simulink model "coord2ASV1UAV"  (R2017a)
settings: Solver=FixedStepAuto  StartTime=0.0  StopTime=720  FixedStep=0.2  RelTol=1e-3
StopFcn:
  | plotVehicles(posHist, tout, start, finish);
settings Model: Creator=acrab  LastModifiedBy=acrab

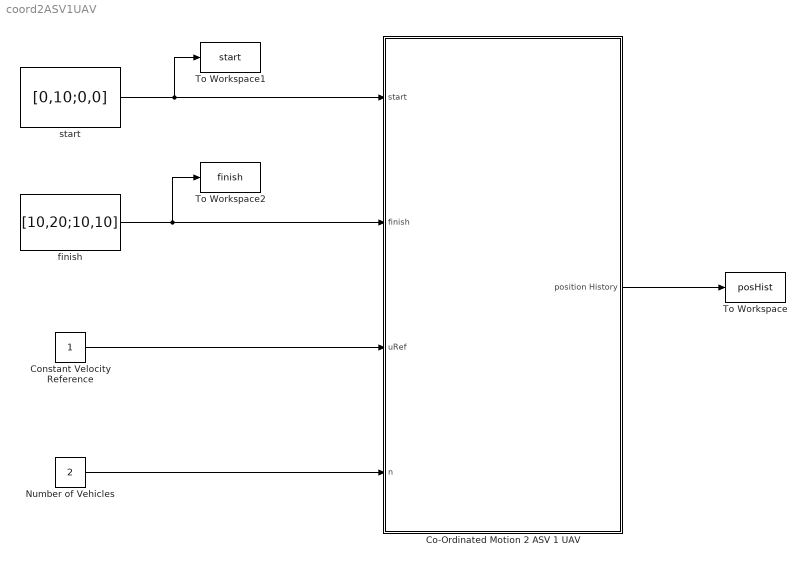
== system coord2ASV1UAV ==
  Co-Ordinated Motion 2 ASV 1 UAV : Subsystem
  Constant Velocity Reference : Constant
  Number of Vehicles : Constant  Value=2
  To Workspace : ToWorkspace  VariableName=posHist  SaveFormat=Structure With Time  SampleTime=-1
  To Workspace1 : ToWorkspace  VariableName=start  SampleTime=-1
  To Workspace2 : ToWorkspace  VariableName=finish  SampleTime=-1
  finish : Constant  Value=[10,20;10,10]
  "start " : Constant  Value=[0,10;0,0]
  wires:
  "start "/1 -> To Workspace1/1, Co-Ordinated Motion 2 ASV 1 UAV/1(start)
  finish/1 -> To Workspace2/1, Co-Ordinated Motion 2 ASV 1 UAV/2(finish)
  Constant Velocity Reference/1 -> Co-Ordinated Motion 2 ASV 1 UAV/3(uRef)
  Number of Vehicles/1 -> Co-Ordinated Motion 2 ASV 1 UAV/4(n)
  Co-Ordinated Motion 2 ASV 1 UAV/1(position History) -> To Workspace/1

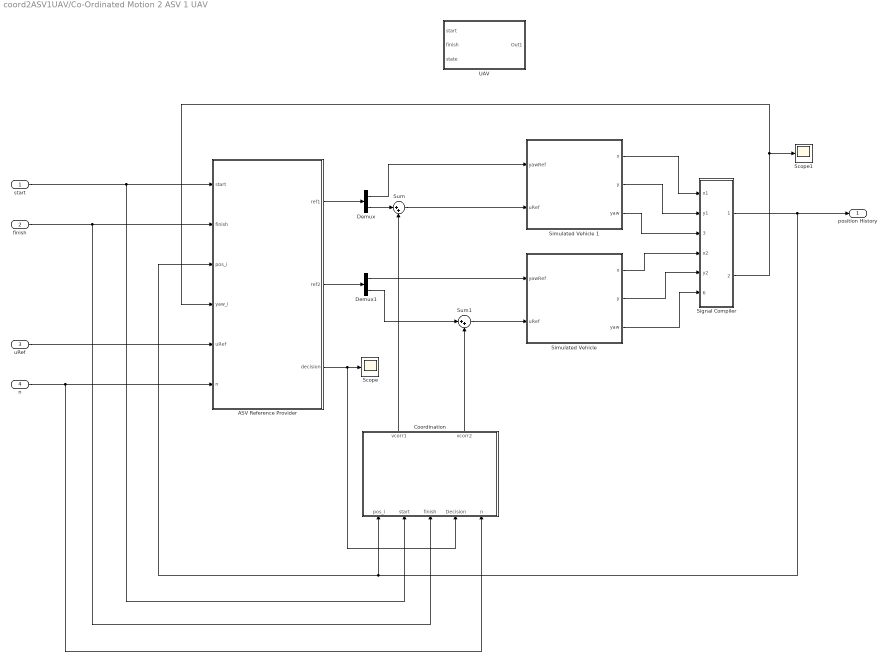
== system coord2ASV1UAV/Co-Ordinated Motion 2 ASV 1 UAV ==
  start : Inport
  finish : Inport  Port=2
  uRef : Inport  Port=3
  n : Inport  Port=4
  ASV Reference Provider : Subsystem
  Coordination : Subsystem  mask{ksync=1, ks=1}
  Demux : Demux  Outputs=2
  Demux1 : Demux  Outputs=2
  Scope : Scope
  Scope1 : Scope
  Signal Compiler : Subsystem
  Simulated Vehicle : Subsystem
  Simulated Vehicle 1 : Subsystem
  Sum : Sum  Inputs=|++
  Sum1 : Sum  Inputs=|++
  UAV : Subsystem
  position History : Outport
  wires:
  Signal Compiler/2(yaw_i) -> Scope1/1, ASV Reference Provider/4(yaw_i)
  Simulated Vehicle 1/3(yaw) -> Signal Compiler/3(yaw1)
  Simulated Vehicle/3(yaw) -> Signal Compiler/6("yaw2 ")
  Sum1/1 -> Simulated Vehicle/2(uRef)
  Demux/1 -> Simulated Vehicle 1/1(yawRef)
  Sum/1 -> Simulated Vehicle 1/2(uRef)
  Demux1/2 -> Sum1/1
  n/1 -> Coordination/5(n), ASV Reference Provider/6("n ")
  Demux1/1 -> Simulated Vehicle/1(yawRef)
  ASV Reference Provider/2("ref2 ") -> Demux1/1
  uRef/1 -> ASV Reference Provider/5(uRef)
  ASV Reference Provider/1(ref1) -> Demux/1
  Simulated Vehicle 1/2(y) -> Signal Compiler/2(y1)
  Coordination/2("vcorr2 ") -> Sum1/2
  Simulated Vehicle 1/1(x) -> Signal Compiler/1(x1)
  ASV Reference Provider/3("decision ") -> Coordination/4(Decision), Scope/1
  start/1 -> ASV Reference Provider/1(start), Coordination/2(start)
  Signal Compiler/1(pos_i) -> position History/1, Coordination/1(pos_i), ASV Reference Provider/3(pos_i)
  Coordination/1(vcorr1) -> Sum/2
  Demux/2 -> Sum/1
  Simulated Vehicle/1(x) -> Signal Compiler/4(x2)
  finish/1 -> ASV Reference Provider/2(finish), Coordination/3(finish)
  Simulated Vehicle/2(y) -> Signal Compiler/5(y2)

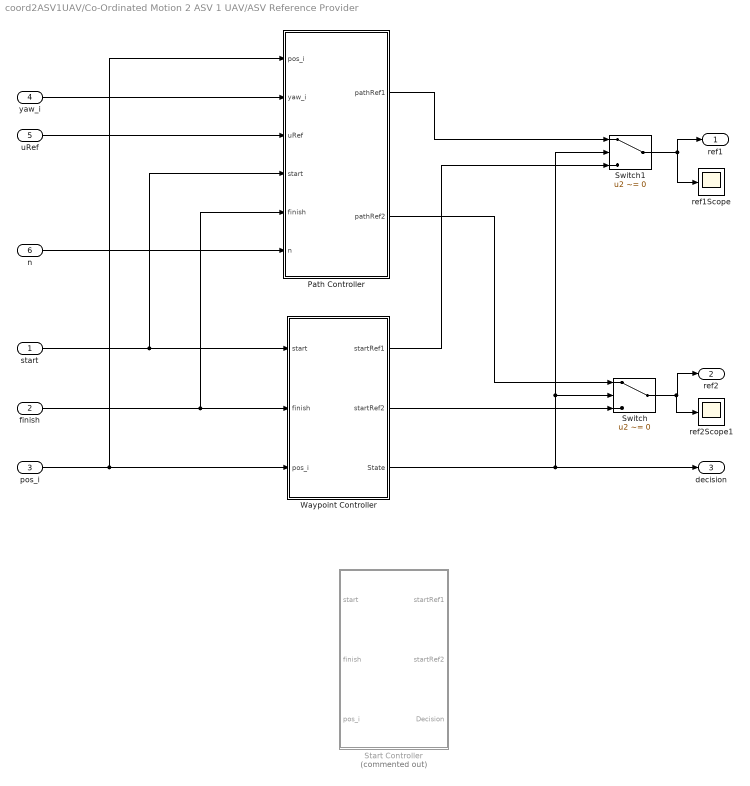
== system coord2ASV1UAV/Co-Ordinated Motion 2 ASV 1 UAV/ASV Reference Provider ==
  start : Inport
  finish : Inport  Port=2
  pos_i : Inport  Port=3
  yaw_i : Inport  Port=4
  uRef : Inport  Port=5
  "n " : Inport  Port=6
  Path Controller : Subsystem
  Start Controller : Subsystem  Commented=on  mask{ku=0.1, ks=0.1}
  Switch : Switch  Criteria=u2 ~= 0  Threshold=0.5
  Switch1 : Switch  Criteria=u2 ~= 0  Threshold=0.5
  Waypoint Controller : Subsystem  mask{ku=0.25, ks=0.1}
  ref1Scope : Scope
  ref2Scope1 : Scope
  ref1 : Outport
  "ref2 " : Outport  Port=2
  "decision " : Outport  Port=3
  wires:
  Waypoint Controller/3(State) -> Switch1/2, Switch/2, "decision "/1
  Waypoint Controller/2(startRef2) -> Switch/3
  Waypoint Controller/1(startRef1) -> Switch1/3
  Switch1/1 -> ref1Scope/1, ref1/1
  Switch/1 -> ref2Scope1/1, "ref2 "/1
  pos_i/1 -> Waypoint Controller/3(pos_i), Path Controller/1(pos_i)
  Path Controller/1(pathRef1) -> Switch1/1
  Path Controller/2(pathRef2) -> Switch/1
  yaw_i/1 -> Path Controller/2(yaw_i)
  uRef/1 -> Path Controller/3(uRef)
  start/1 -> Path Controller/4(start), Waypoint Controller/1("start ")
  finish/1 -> Waypoint Controller/2(finish), Path Controller/5(finish)
  "n "/1 -> Path Controller/6(n)

== system coord2ASV1UAV/Co-Ordinated Motion 2 ASV 1 UAV/Coordination ==
  pos_i : Inport
  start : Inport  Port=2
  finish : Inport  Port=3
  Decision : Inport  Port=4
  n : Inport  Port=5
  Co-Ordination Controller : MATLAB Function  TreatAsAtomicUnit=on
  Constant : Constant  Value=0
  vcorr1 : Outport
  "vcorr2 " : Outport  Port=2
  wires:
  n/1 -> Co-Ordination Controller/1(n)
  pos_i/1 -> Co-Ordination Controller/2(pos_i)
  start/1 -> Co-Ordination Controller/3(start)
  finish/1 -> Co-Ordination Controller/4(finish)
  Constant/1 -> Co-Ordination Controller/5(pathType)
  Co-Ordination Controller/1(vcorr1) -> vcorr1/1
  Co-Ordination Controller/2(vcorr2) -> "vcorr2 "/1
  Decision/1 -> Co-Ordination Controller/6(decision)

== system coord2ASV1UAV/Co-Ordinated Motion 2 ASV 1 UAV/Signal Compiler ==
  x1 : Inport
  y1 : Inport  Port=2
  yaw1 : Inport  Port=3
  x2 : Inport  Port=4
  y2 : Inport  Port=5
  "yaw2 " : Inport  Port=6
  MATLAB Function : MATLAB Function  TreatAsAtomicUnit=on
  pos_i : Outport
  yaw_i : Outport  Port=2
  wires:
  x2/1 -> MATLAB Function/4(x2)
  y2/1 -> MATLAB Function/5(y2)
  y1/1 -> MATLAB Function/2(y1)
  x1/1 -> MATLAB Function/1(x1)
  MATLAB Function/1(pos_i) -> pos_i/1
  yaw1/1 -> MATLAB Function/3(yaw1)
  "yaw2 "/1 -> MATLAB Function/6(yaw2)
  MATLAB Function/2(yaw_i) -> yaw_i/1

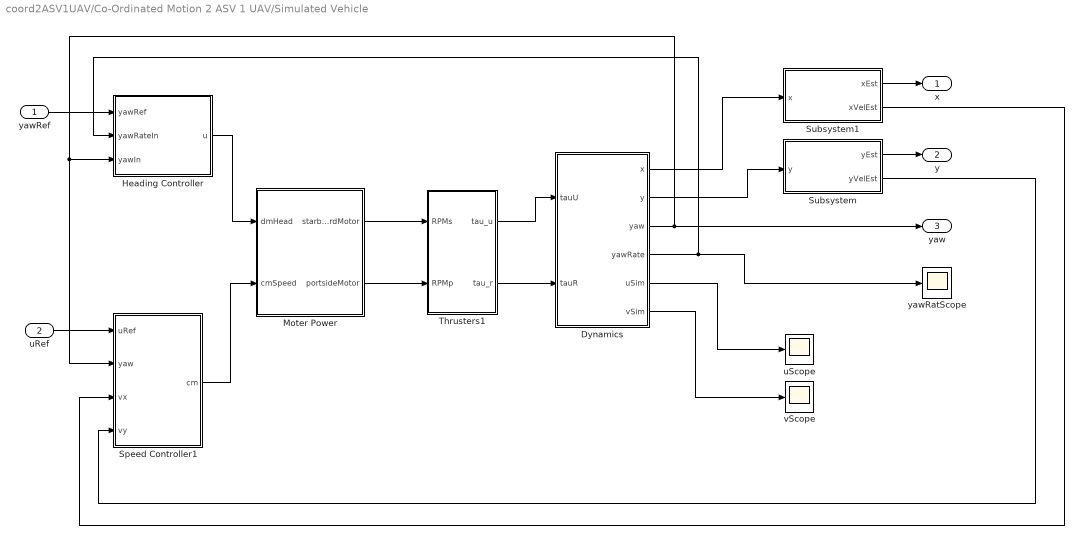
== system coord2ASV1UAV/Co-Ordinated Motion 2 ASV 1 UAV/Simulated Vehicle ==
  yawRef : Inport
  uRef : Inport  Port=2
  Dynamics : Subsystem
  Heading Controller : Subsystem  mask{Kp=45, Kd=110}
  Moter Power : Subsystem
  Speed Controller1 : Subsystem  mask{Kp=60, Ki=2, KSat=60}
      mask prompts: KSat "Saturation Level"
  Subsystem : Subsystem
  Subsystem1 : Subsystem
  Thrusters1 : Subsystem
  uScope : Scope
  vScope : Scope
  yawRatScope : Scope
  x : Outport
  y : Outport  Port=2
  yaw : Outport  Port=3
  wires:
  Thrusters1/1(tau_u) -> Dynamics/1(tauU)
  Thrusters1/2(tau_r) -> Dynamics/2(tauR)
  Moter Power/1(starboardMotor) -> Thrusters1/1(RPMs)
  Moter Power/2(portsideMotor) -> Thrusters1/2(RPMp)
  Dynamics/3(yaw) -> Speed Controller1/2(yaw), Heading Controller/3(yawIn), yaw/1
  Dynamics/4(yawRate) -> yawRatScope/1, Heading Controller/2(yawRateIn)
  Dynamics/5(uSim) -> uScope/1
  Dynamics/6(vSim) -> vScope/1
  yawRef/1 -> Heading Controller/1(yawRef)
  uRef/1 -> Speed Controller1/1(uRef)
  Subsystem/1(yEst) -> y/1
  Dynamics/2(y) -> Subsystem/1(y)
  Heading Controller/1(u) -> Moter Power/1(dmHead)
  Speed Controller1/1(cm) -> Moter Power/2(cmSpeed)
  Dynamics/1(x) -> Subsystem1/1(x)
  Subsystem1/1(xEst) -> x/1
  Subsystem/2(yVelEst) -> Speed Controller1/4(vy)
  Subsystem1/2(xVelEst) -> Speed Controller1/3(vx)

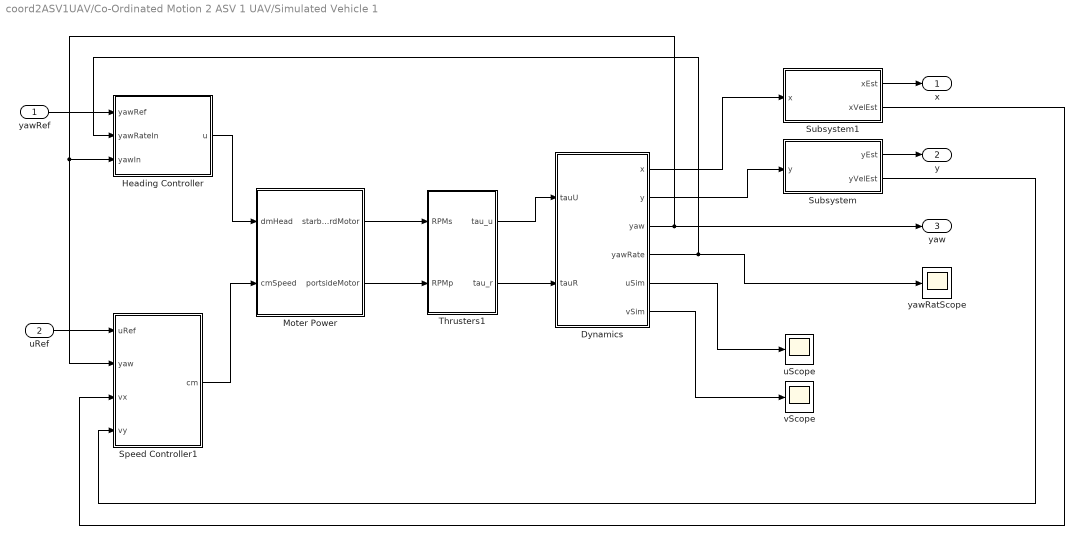
== system coord2ASV1UAV/Co-Ordinated Motion 2 ASV 1 UAV/Simulated Vehicle 1 ==
  yawRef : Inport
  uRef : Inport  Port=2
  Dynamics : Subsystem
  Heading Controller : Subsystem  mask{Kp=45, Kd=110}
  Moter Power : Subsystem
  Speed Controller1 : Subsystem  mask{Kp=60, Ki=2, KSat=60}
      mask prompts: KSat "Saturation Level"
  Subsystem : Subsystem
  Subsystem1 : Subsystem
  Thrusters1 : Subsystem
  uScope : Scope
  vScope : Scope
  yawRatScope : Scope
  x : Outport
  y : Outport  Port=2
  yaw : Outport  Port=3
  wires:
  Thrusters1/1(tau_u) -> Dynamics/1(tauU)
  Thrusters1/2(tau_r) -> Dynamics/2(tauR)
  Moter Power/1(starboardMotor) -> Thrusters1/1(RPMs)
  Moter Power/2(portsideMotor) -> Thrusters1/2(RPMp)
  Dynamics/3(yaw) -> Speed Controller1/2(yaw), Heading Controller/3(yawIn), yaw/1
  Dynamics/4(yawRate) -> yawRatScope/1, Heading Controller/2(yawRateIn)
  Dynamics/5(uSim) -> uScope/1
  Dynamics/6(vSim) -> vScope/1
  yawRef/1 -> Heading Controller/1(yawRef)
  uRef/1 -> Speed Controller1/1(uRef)
  Subsystem/1(yEst) -> y/1
  Dynamics/2(y) -> Subsystem/1(y)
  Heading Controller/1(u) -> Moter Power/1(dmHead)
  Speed Controller1/1(cm) -> Moter Power/2(cmSpeed)
  Dynamics/1(x) -> Subsystem1/1(x)
  Subsystem1/1(xEst) -> x/1
  Subsystem/2(yVelEst) -> Speed Controller1/4(vy)
  Subsystem1/2(xVelEst) -> Speed Controller1/3(vx)

== system coord2ASV1UAV/Co-Ordinated Motion 2 ASV 1 UAV/UAV ==
  start : Inport
  finish : Inport  Port=2
  state : Inport  Port=3
  Out1 : Outport

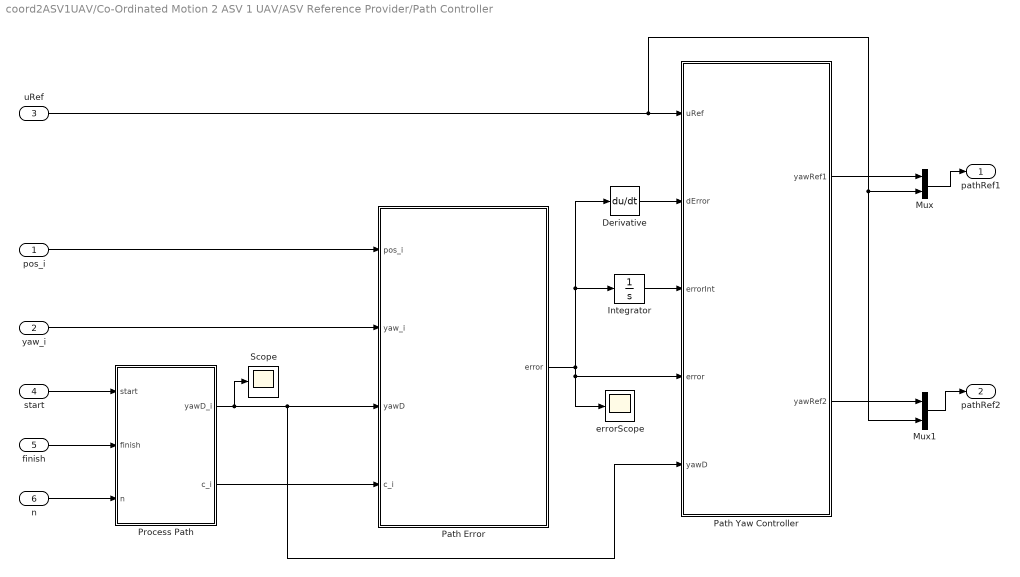
== system coord2ASV1UAV/Co-Ordinated Motion 2 ASV 1 UAV/ASV Reference Provider/Path Controller ==
  pos_i : Inport
  yaw_i : Inport  Port=2
  uRef : Inport  Port=3
  start : Inport  Port=4
  finish : Inport  Port=5
  n : Inport  Port=6
  Derivative : Derivative
  Integrator : Integrator
  Mux : Mux  Inputs=2
  Mux1 : Mux  Inputs=2
  Path Error : MATLAB Function  TreatAsAtomicUnit=on
  Path Yaw Controller : MATLAB Function  TreatAsAtomicUnit=on
  Process Path : MATLAB Function  TreatAsAtomicUnit=on
  Scope : Scope
  errorScope : Scope
  pathRef1 : Outport
  pathRef2 : Outport  Port=2
  wires:
  start/1 -> Process Path/1(start)
  Derivative/1 -> Path Yaw Controller/2(dError)
  uRef/1 -> Mux1/2, Mux/2, Path Yaw Controller/1(uRef)
  yaw_i/1 -> Path Error/2(yaw_i)
  Process Path/1(yawD_i) -> Scope/1, Path Yaw Controller/5(yawD), Path Error/3(yawD)
  Path Error/1(error) -> errorScope/1, Path Yaw Controller/4(error), Integrator/1, Derivative/1
  Process Path/2(c_i) -> Path Error/4(c_i)
  pos_i/1 -> Path Error/1(pos_i)
  n/1 -> Process Path/3(n)
  finish/1 -> Process Path/2(finish)
  Mux/1 -> pathRef1/1
  Mux1/1 -> pathRef2/1
  Path Yaw Controller/1(yawRef1) -> Mux/1
  Path Yaw Controller/2(yawRef2) -> Mux1/1
  Integrator/1 -> Path Yaw Controller/3(errorInt)

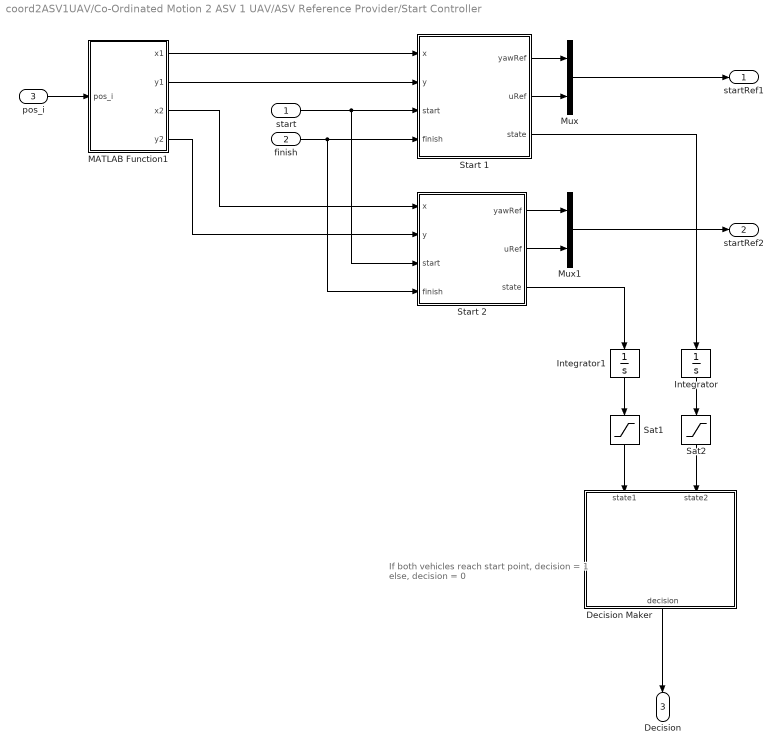
== system coord2ASV1UAV/Co-Ordinated Motion 2 ASV 1 UAV/ASV Reference Provider/Start Controller ==
  note: If both vehicles reach start point, decision = 1
      | else, decision = 0
  start : Inport
  finish : Inport  Port=2
  "pos_i " : Inport  Port=3
  Decision Maker : MATLAB Function  TreatAsAtomicUnit=on
  Integrator : Integrator
  Integrator1 : Integrator
  MATLAB Function1 : MATLAB Function  TreatAsAtomicUnit=on
  Mux : Mux  Inputs=2
  Mux1 : Mux  Inputs=2
  Sat1 : Saturate  UpperLimit=1  LowerLimit=0
  Sat2 : Saturate  UpperLimit=1  LowerLimit=0
  Start 1 : MATLAB Function  TreatAsAtomicUnit=on
  Start 2 : MATLAB Function  TreatAsAtomicUnit=on
  startRef1 : Outport
  startRef2 : Outport  Port=2
  Decision : Outport  Port=3
  wires:
  MATLAB Function1/2(y1) -> Start 1/2(y)
  start/1 -> Start 2/3(start), Start 1/3(start)
  MATLAB Function1/1(x1) -> Start 1/1(x)
  finish/1 -> Start 2/4(finish), Start 1/4(finish)
  MATLAB Function1/3(x2) -> Start 2/1(x)
  MATLAB Function1/4(y2) -> Start 2/2(y)
  Start 1/1(yawRef) -> Mux/1
  Start 1/2(uRef) -> Mux/2
  Mux/1 -> startRef1/1
  Start 2/1(yawRef) -> Mux1/1
  Start 2/2(uRef) -> Mux1/2
  Mux1/1 -> startRef2/1
  "pos_i "/1 -> MATLAB Function1/1(pos_i)
  Start 1/3(state) -> Integrator/1
  Start 2/3(state) -> Integrator1/1
  Sat1/1 -> Decision Maker/1(state1)
  Integrator1/1 -> Sat1/1
  Integrator/1 -> Sat2/1
  Sat2/1 -> Decision Maker/2(state2)
  Decision Maker/1(decision) -> Decision/1

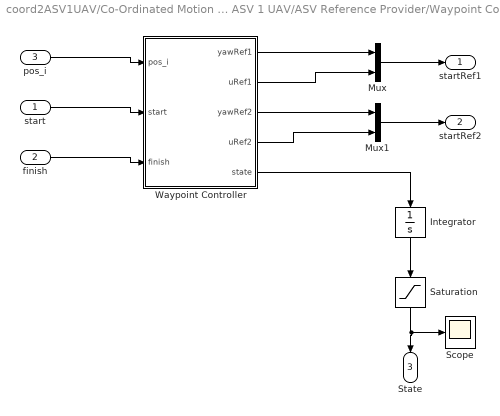
== system coord2ASV1UAV/Co-Ordinated Motion 2 ASV 1 UAV/ASV Reference Provider/Waypoint Controller ==
  "start " : Inport
  finish : Inport  Port=2
  pos_i : Inport  Port=3
  Integrator : Integrator
  Mux : Mux  Inputs=2
  Mux1 : Mux  Inputs=2
  Saturation : Saturate  UpperLimit=1  LowerLimit=0
  Scope : Scope
  Waypoint Controller : MATLAB Function  TreatAsAtomicUnit=on
  startRef1 : Outport
  startRef2 : Outport  Port=2
  State : Outport  Port=3
  wires:
  pos_i/1 -> Waypoint Controller/1(pos_i)
  "start "/1 -> Waypoint Controller/2(start)
  finish/1 -> Waypoint Controller/3(finish)
  Waypoint Controller/5(state) -> Integrator/1
  Integrator/1 -> Saturation/1
  Saturation/1 -> State/1, Scope/1
  Waypoint Controller/1(yawRef1) -> Mux/1
  Waypoint Controller/2(uRef1) -> Mux/2
  Mux/1 -> startRef1/1
  Waypoint Controller/3(yawRef2) -> Mux1/1
  Waypoint Controller/4(uRef2) -> Mux1/2
  Mux1/1 -> startRef2/1

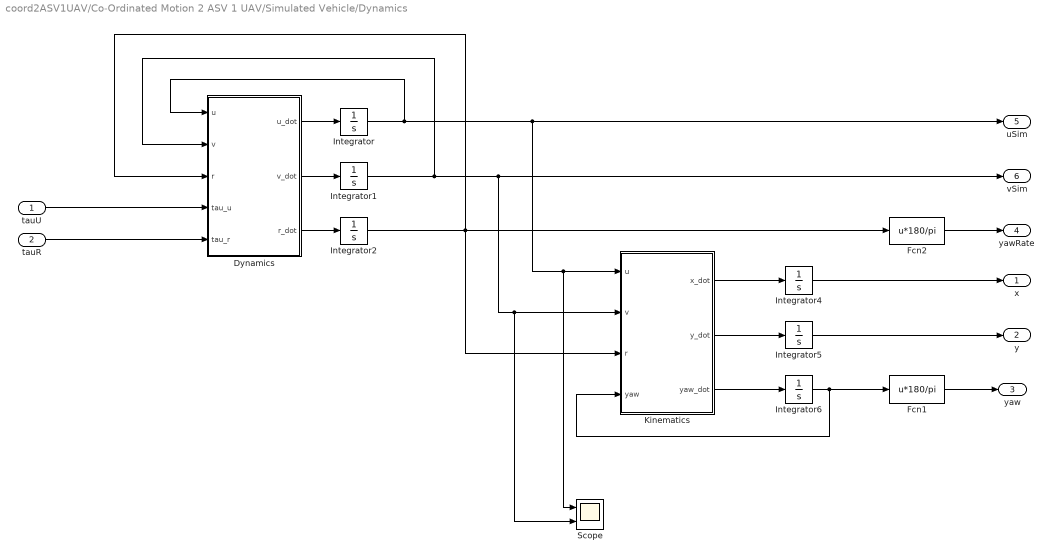
== system coord2ASV1UAV/Co-Ordinated Motion 2 ASV 1 UAV/Simulated Vehicle/Dynamics ==
  tauU : Inport
  tauR : Inport  Port=2
  Dynamics : MATLAB Function  TreatAsAtomicUnit=on
  Fcn1 : Fcn  Expr=u*180/pi
  Fcn2 : Fcn  Expr=u*180/pi
  Integrator{,1..2,4..6} (6 alike) : Integrator
  Kinematics : MATLAB Function  TreatAsAtomicUnit=on
  Scope : Scope  NumInputPorts=2
  x : Outport
  y : Outport  Port=2
  yaw : Outport  Port=3
  yawRate : Outport  Port=4
  uSim : Outport  Port=5
  vSim : Outport  Port=6
  wires:
  tauR/1 -> Dynamics/5(tau_r)
  tauU/1 -> Dynamics/4(tau_u)
  Dynamics/1(u_dot) -> Integrator/1
  Dynamics/3(r_dot) -> Integrator2/1
  Dynamics/2(v_dot) -> Integrator1/1
  Kinematics/1(x_dot) -> Integrator4/1
  Kinematics/2(y_dot) -> Integrator5/1
  Kinematics/3(yaw_dot) -> Integrator6/1
  Integrator/1 -> uSim/1, Scope/1, Kinematics/1(u), Dynamics/1(u)
  Integrator1/1 -> vSim/1, Kinematics/2(v), Scope/2, Dynamics/2(v)
  Integrator2/1 -> Fcn2/1, Kinematics/3(r), Dynamics/3(r)
  Integrator4/1 -> x/1
  Integrator5/1 -> y/1
  Integrator6/1 -> Fcn1/1, Kinematics/4(yaw)
  Fcn1/1 -> yaw/1
  Fcn2/1 -> yawRate/1

== system coord2ASV1UAV/Co-Ordinated Motion 2 ASV 1 UAV/Simulated Vehicle/Heading Controller ==
  yawRef : Inport
  yawRateIn : Inport  Port=2
  yawIn : Inport  Port=3
  Kd : Gain  Gain=Kd
  Kp : Gain  Gain=Kp
  MATLAB Function : MATLAB Function  TreatAsAtomicUnit=on
  Sum1 : Sum  Inputs=|+-
  u : Outport
  wires:
  yawRef/1 -> MATLAB Function/1(yawRef)
  yawRateIn/1 -> Kd/1
  Kd/1 -> Sum1/2
  Kp/1 -> Sum1/1
  Sum1/1 -> u/1
  MATLAB Function/1(err) -> Kp/1
  yawIn/1 -> MATLAB Function/2(yawIn)

== system coord2ASV1UAV/Co-Ordinated Motion 2 ASV 1 UAV/Simulated Vehicle/Moter Power ==
  dmHead : Inport
  cmSpeed : Inport  Port=2
  MATLAB Function : MATLAB Function  TreatAsAtomicUnit=on
  starboardMotor : Outport
  portsideMotor : Outport  Port=2
  wires:
  dmHead/1 -> MATLAB Function/1(dmHead)
  cmSpeed/1 -> MATLAB Function/2(cmSpeed)
  MATLAB Function/1(Pm) -> portsideMotor/1
  MATLAB Function/2(Sm) -> starboardMotor/1

== system coord2ASV1UAV/Co-Ordinated Motion 2 ASV 1 UAV/Simulated Vehicle/Speed Controller1 ==
  uRef : Inport
  yaw : Inport  Port=2
  vx : Inport  Port=3
  vy : Inport  Port=4
  Unit Delay : UnitDelay  SampleTime=-1
  sqr : Fcn  Expr=abs(u)*u
  u Speed from Estimates : MATLAB Function  TreatAsAtomicUnit=on
  cm : Outport
  wires:
  vx/1 -> u Speed from Estimates/1(vx)
  yaw/1 -> u Speed from Estimates/3(yaw)
  vy/1 -> u Speed from Estimates/2(vy)
  uRef/1 -> u Speed from Estimates/4(Uref)
  sqr/1 -> cm/1
  Unit Delay/1 -> u Speed from Estimates/5(intOld)
  u Speed from Estimates/1(cm) -> sqr/1
  u Speed from Estimates/2(int) -> Unit Delay/1

== system coord2ASV1UAV/Co-Ordinated Motion 2 ASV 1 UAV/Simulated Vehicle/Subsystem ==
  y : Inport
  Derivative : Derivative
  yEst : Outport
  yVelEst : Outport  Port=2
  wires:
  y/1 -> Derivative/1, yEst/1
  Derivative/1 -> yVelEst/1

== system coord2ASV1UAV/Co-Ordinated Motion 2 ASV 1 UAV/Simulated Vehicle/Subsystem1 ==
  x : Inport
  Derivative : Derivative
  xEst : Outport
  xVelEst : Outport  Port=2
  wires:
  x/1 -> Derivative/1, xEst/1
  Derivative/1 -> xVelEst/1

== system coord2ASV1UAV/Co-Ordinated Motion 2 ASV 1 UAV/Simulated Vehicle/Thrusters1 ==
  RPMs : Inport
  RPMp : Inport  Port=2
  Add : Sum
  Add1 : Sum  Inputs=-+
  Motor Port : Subsystem  mask{K0=7.2115, tau=0.346, eta=4/(1500^2)}
      mask prompts: tau "Atraso do Motor"; eta "Constante de conversao W-F"
  Motor Stardboard : Subsystem  mask{K0=7.2115, tau=0.346, eta=4/(1500^2)}
      mask prompts: tau "Atraso do Motor"; eta "Constante de conversao W-F"
  l : Gain  Gain=0.25
  tau_u : Outport
  tau_r : Outport  Port=2
  wires:
  Add1/1 -> l/1
  RPMs/1 -> Motor Stardboard/1(w RPM)
  Add/1 -> tau_u/1
  RPMp/1 -> Motor Port/1(w RPM)
  l/1 -> tau_r/1
  Motor Port/1(F) -> Add/2, Add1/2
  Motor Stardboard/1(F) -> Add/1, Add1/1

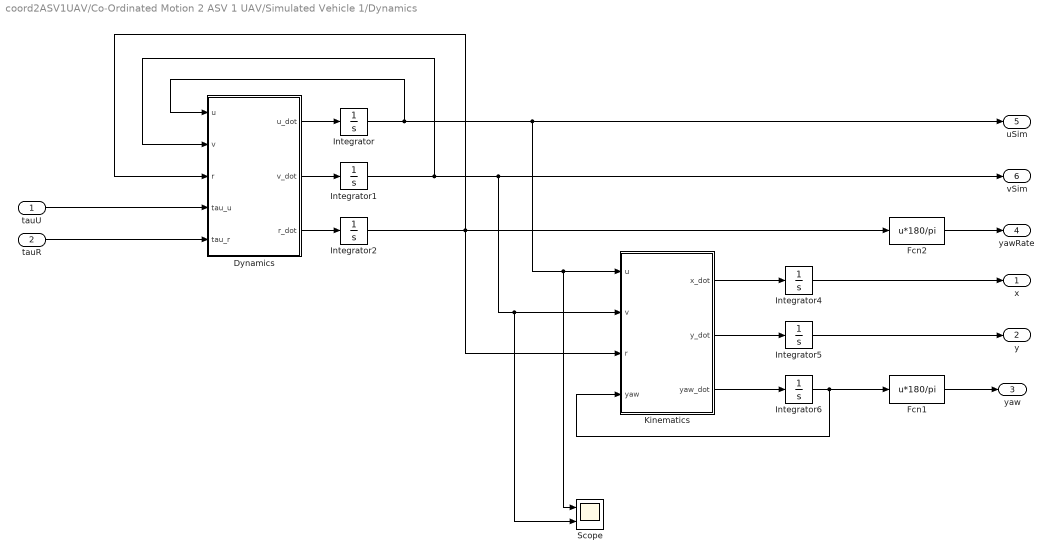
== system coord2ASV1UAV/Co-Ordinated Motion 2 ASV 1 UAV/Simulated Vehicle 1/Dynamics ==
  tauU : Inport
  tauR : Inport  Port=2
  Dynamics : MATLAB Function  TreatAsAtomicUnit=on
  Fcn1 : Fcn  Expr=u*180/pi
  Fcn2 : Fcn  Expr=u*180/pi
  Integrator{,1..2,4..6} (6 alike) : Integrator
  Kinematics : MATLAB Function  TreatAsAtomicUnit=on
  Scope : Scope  NumInputPorts=2
  x : Outport
  y : Outport  Port=2
  yaw : Outport  Port=3
  yawRate : Outport  Port=4
  uSim : Outport  Port=5
  vSim : Outport  Port=6
  wires:
  tauR/1 -> Dynamics/5(tau_r)
  tauU/1 -> Dynamics/4(tau_u)
  Dynamics/1(u_dot) -> Integrator/1
  Dynamics/3(r_dot) -> Integrator2/1
  Dynamics/2(v_dot) -> Integrator1/1
  Kinematics/1(x_dot) -> Integrator4/1
  Kinematics/2(y_dot) -> Integrator5/1
  Kinematics/3(yaw_dot) -> Integrator6/1
  Integrator/1 -> uSim/1, Scope/1, Kinematics/1(u), Dynamics/1(u)
  Integrator1/1 -> vSim/1, Kinematics/2(v), Scope/2, Dynamics/2(v)
  Integrator2/1 -> Fcn2/1, Kinematics/3(r), Dynamics/3(r)
  Integrator4/1 -> x/1
  Integrator5/1 -> y/1
  Integrator6/1 -> Fcn1/1, Kinematics/4(yaw)
  Fcn1/1 -> yaw/1
  Fcn2/1 -> yawRate/1

== system coord2ASV1UAV/Co-Ordinated Motion 2 ASV 1 UAV/Simulated Vehicle 1/Heading Controller ==
  yawRef : Inport
  yawRateIn : Inport  Port=2
  yawIn : Inport  Port=3
  Kd : Gain  Gain=Kd
  Kp : Gain  Gain=Kp
  MATLAB Function : MATLAB Function  TreatAsAtomicUnit=on
  Sum1 : Sum  Inputs=|+-
  u : Outport
  wires:
  yawRef/1 -> MATLAB Function/1(yawRef)
  yawRateIn/1 -> Kd/1
  Kd/1 -> Sum1/2
  Kp/1 -> Sum1/1
  Sum1/1 -> u/1
  MATLAB Function/1(err) -> Kp/1
  yawIn/1 -> MATLAB Function/2(yawIn)

== system coord2ASV1UAV/Co-Ordinated Motion 2 ASV 1 UAV/Simulated Vehicle 1/Moter Power ==
  dmHead : Inport
  cmSpeed : Inport  Port=2
  MATLAB Function : MATLAB Function  TreatAsAtomicUnit=on
  starboardMotor : Outport
  portsideMotor : Outport  Port=2
  wires:
  dmHead/1 -> MATLAB Function/1(dmHead)
  cmSpeed/1 -> MATLAB Function/2(cmSpeed)
  MATLAB Function/1(Pm) -> portsideMotor/1
  MATLAB Function/2(Sm) -> starboardMotor/1

== system coord2ASV1UAV/Co-Ordinated Motion 2 ASV 1 UAV/Simulated Vehicle 1/Speed Controller1 ==
  uRef : Inport
  yaw : Inport  Port=2
  vx : Inport  Port=3
  vy : Inport  Port=4
  Unit Delay : UnitDelay  SampleTime=-1
  sqr : Fcn  Expr=abs(u)*u
  u Speed from Estimates : MATLAB Function  TreatAsAtomicUnit=on
  cm : Outport
  wires:
  vx/1 -> u Speed from Estimates/1(vx)
  yaw/1 -> u Speed from Estimates/3(yaw)
  vy/1 -> u Speed from Estimates/2(vy)
  uRef/1 -> u Speed from Estimates/4(Uref)
  sqr/1 -> cm/1
  Unit Delay/1 -> u Speed from Estimates/5(intOld)
  u Speed from Estimates/1(cm) -> sqr/1
  u Speed from Estimates/2(int) -> Unit Delay/1

== system coord2ASV1UAV/Co-Ordinated Motion 2 ASV 1 UAV/Simulated Vehicle 1/Subsystem ==
  y : Inport
  Derivative : Derivative
  yEst : Outport
  yVelEst : Outport  Port=2
  wires:
  y/1 -> Derivative/1, yEst/1
  Derivative/1 -> yVelEst/1

== system coord2ASV1UAV/Co-Ordinated Motion 2 ASV 1 UAV/Simulated Vehicle 1/Subsystem1 ==
  x : Inport
  Derivative : Derivative
  xEst : Outport
  xVelEst : Outport  Port=2
  wires:
  x/1 -> Derivative/1, xEst/1
  Derivative/1 -> xVelEst/1

== system coord2ASV1UAV/Co-Ordinated Motion 2 ASV 1 UAV/Simulated Vehicle 1/Thrusters1 ==
  RPMs : Inport
  RPMp : Inport  Port=2
  Add : Sum
  Add1 : Sum  Inputs=-+
  Motor Port : Subsystem  mask{K0=7.2115, tau=0.346, eta=4/(1500^2)}
      mask prompts: tau "Atraso do Motor"; eta "Constante de conversao W-F"
  Motor Stardboard : Subsystem  mask{K0=7.2115, tau=0.346, eta=4/(1500^2)}
      mask prompts: tau "Atraso do Motor"; eta "Constante de conversao W-F"
  l : Gain  Gain=0.25
  tau_u : Outport
  tau_r : Outport  Port=2
  wires:
  Add1/1 -> l/1
  RPMs/1 -> Motor Stardboard/1(w RPM)
  Add/1 -> tau_u/1
  RPMp/1 -> Motor Port/1(w RPM)
  l/1 -> tau_r/1
  Motor Port/1(F) -> Add/2, Add1/2
  Motor Stardboard/1(F) -> Add/1, Add1/1

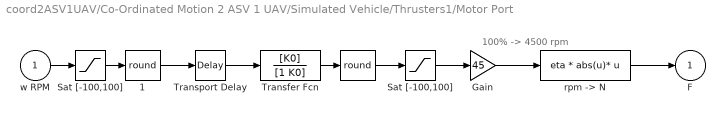
== system coord2ASV1UAV/Co-Ordinated Motion 2 ASV 1 UAV/Simulated Vehicle/Thrusters1/Motor Port ==
  note: 100% -> 4500 rpm
  w RPM : Inport
  "  " : Rounding  Operator=round
  "  1" : Rounding  Operator=round
  Gain : Gain  Gain=45
  Sat [-100,100] : Saturate  UpperLimit=100  LowerLimit=-100
  "Sat [-100,100] " : Saturate  UpperLimit=100  LowerLimit=-100
  Transfer Fcn : TransferFcn  Numerator=[K0]  Denominator=[1 K0]
  Transport Delay : TransportDelay  DelayTime=tau
  "rpm -> N" : Fcn  Expr=eta * abs(u)* u
  F : Outport
  wires:
  Transfer Fcn/1 -> "  "/1
  Transport Delay/1 -> Transfer Fcn/1
  "  1"/1 -> Transport Delay/1
  "  "/1 -> "Sat [-100,100] "/1
  "rpm -> N"/1 -> F/1
  Sat [-100,100]/1 -> "  1"/1
  Gain/1 -> "rpm -> N"/1
  w RPM/1 -> Sat [-100,100]/1
  "Sat [-100,100] "/1 -> Gain/1

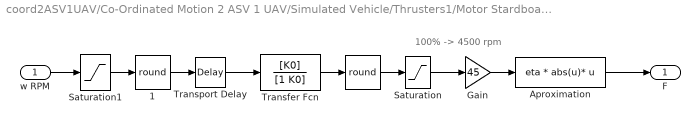
== system coord2ASV1UAV/Co-Ordinated Motion 2 ASV 1 UAV/Simulated Vehicle/Thrusters1/Motor Stardboard ==
  note: 100% -> 4500 rpm
  w RPM : Inport
  "  " : Rounding  Operator=round
  "  1" : Rounding  Operator=round
  Aproximation : Fcn  Expr=eta * abs(u)* u
  Gain : Gain  Gain=45
  Saturation : Saturate  UpperLimit=100  LowerLimit=-100
  Saturation1 : Saturate  UpperLimit=100  LowerLimit=-100
  Transfer Fcn : TransferFcn  Numerator=[K0]  Denominator=[1 K0]
  Transport Delay : TransportDelay  DelayTime=tau
  F : Outport
  wires:
  Transfer Fcn/1 -> "  "/1
  Transport Delay/1 -> Transfer Fcn/1
  "  1"/1 -> Transport Delay/1
  "  "/1 -> Saturation/1
  Aproximation/1 -> F/1
  Saturation1/1 -> "  1"/1
  Gain/1 -> Aproximation/1
  w RPM/1 -> Saturation1/1
  Saturation/1 -> Gain/1

== system coord2ASV1UAV/Co-Ordinated Motion 2 ASV 1 UAV/Simulated Vehicle 1/Thrusters1/Motor Port ==
  note: 100% -> 4500 rpm
  w RPM : Inport
  "  " : Rounding  Operator=round
  "  1" : Rounding  Operator=round
  Gain : Gain  Gain=45
  Sat [-100,100] : Saturate  UpperLimit=100  LowerLimit=-100
  "Sat [-100,100] " : Saturate  UpperLimit=100  LowerLimit=-100
  Transfer Fcn : TransferFcn  Numerator=[K0]  Denominator=[1 K0]
  Transport Delay : TransportDelay  DelayTime=tau
  "rpm -> N" : Fcn  Expr=eta * abs(u)* u
  F : Outport
  wires:
  Transfer Fcn/1 -> "  "/1
  Transport Delay/1 -> Transfer Fcn/1
  "  1"/1 -> Transport Delay/1
  "  "/1 -> "Sat [-100,100] "/1
  "rpm -> N"/1 -> F/1
  Sat [-100,100]/1 -> "  1"/1
  Gain/1 -> "rpm -> N"/1
  w RPM/1 -> Sat [-100,100]/1
  "Sat [-100,100] "/1 -> Gain/1

== system coord2ASV1UAV/Co-Ordinated Motion 2 ASV 1 UAV/Simulated Vehicle 1/Thrusters1/Motor Stardboard ==
  note: 100% -> 4500 rpm
  w RPM : Inport
  "  " : Rounding  Operator=round
  "  1" : Rounding  Operator=round
  Aproximation : Fcn  Expr=eta * abs(u)* u
  Gain : Gain  Gain=45
  Saturation : Saturate  UpperLimit=100  LowerLimit=-100
  Saturation1 : Saturate  UpperLimit=100  LowerLimit=-100
  Transfer Fcn : TransferFcn  Numerator=[K0]  Denominator=[1 K0]
  Transport Delay : TransportDelay  DelayTime=tau
  F : Outport
  wires:
  Transfer Fcn/1 -> "  "/1
  Transport Delay/1 -> Transfer Fcn/1
  "  1"/1 -> Transport Delay/1
  "  "/1 -> Saturation/1
  Aproximation/1 -> F/1
  Saturation1/1 -> "  1"/1
  Gain/1 -> Aproximation/1
  w RPM/1 -> Saturation1/1
  Saturation/1 -> Gain/1

== matlab function coord2ASV1UAV/Co-Ordinated Motion 2 ASV 1 UAV/Simulated Vehicle 1/Dynamics/Dynamics ==
  data: u input; u_dot output; v input; r input; tau_u input; tau_r input; v_dot output; r_dot output
function [u_dot,v_dot,r_dot] = fcn(u,v,r,tau_u,tau_r)

% Coefficients
m = 17; %kg
Iz = 1; %4.14;
X_u_dot = -20;
Y_v_dot = -30;%-1.3175;
N_r_dot = -8.69;% -0.5;
X_u = -0.2;
Y_v = -50; %-55.117;
N_r = -4.14; %-0.1
X_uu = -25;
Y_vv = -0.01;%-101.2776;
N_rr = -6.23; %-21

% Added Mass
mu = m - X_u_dot;
mv = m - Y_v_dot;
mr = Iz - N_r_dot;
muv = mu - mv;

% Hydrodynamic Damping
du = - X_u - X_uu*abs(u);
dv = - Y_v - Y_vv*abs(v);
dr = - N_r - N_rr*abs(r);

% State Derivatives
u_dot = 1/mu*(tau_u + mv*v*r - du*u);
v_dot = 1/mv*(- mu*u*r - dv*v);
r_dot = 1/mr*(tau_r + muv*u*v - dr*r);

== matlab function coord2ASV1UAV/Co-Ordinated Motion 2 ASV 1 UAV/Simulated Vehicle 1/Speed Controller1/u Speed from Estimates ==
  data: vx input; cm output; vy input; yaw input; Uref input; int output; intOld input; Kp parameter; Ki parameter; KSat parameter
function [cm,int] = ExtractSpeed(vx,vy,yaw,Uref,intOld,Kp, Ki, KSat)

% Kp = 60;
% Ki = 2;
% KSat = 60;
 
u = vx*sind(yaw) + vy*cosd(yaw);
err = u - Uref;
int = intOld + err;

cm = - Kp*err - Ki*int;

if(abs(cm) >= KSat)
   cm = KSat*sign(cm); 
   int = intOld;
end

== matlab function coord2ASV1UAV/Co-Ordinated Motion 2 ASV 1 UAV/Simulated Vehicle 1/Dynamics/Kinematics ==
  data: u input; x_dot output; v input; r input; yaw input; y_dot output; yaw_dot output
function [x_dot,y_dot,yaw_dot] = fcn(u,v,r,yaw)

y_dot = u*cos(yaw) - v*sin(yaw);
x_dot = u*sin(yaw) + v*cos(yaw);
yaw_dot = r;

== matlab function coord2ASV1UAV/Co-Ordinated Motion 2 ASV 1 UAV/Simulated Vehicle 1/Moter Power/MATLAB Function ==
  data: dmHead input; cmSpeed input; Pm output; Sm output
function [Pm,Sm] = fcn(dmHead,cmSpeed)

Cm_sqr = cmSpeed;
Dm_sqr = dmHead;

Pm = round(sqrt(abs(Cm_sqr+Dm_sqr))*sign(Cm_sqr+Dm_sqr));
Sm = round(sqrt(abs(Cm_sqr-Dm_sqr))*sign(Cm_sqr-Dm_sqr));

== matlab function coord2ASV1UAV/Co-Ordinated Motion 2 ASV 1 UAV/Simulated Vehicle 1/Heading Controller/MATLAB Function ==
  data: err output; yawRef input; yawIn input
function err = fcn(yawRef,yawIn)
%error term
err = yawRef - yawIn;

%normalize
if(err>180) 
     err = err - 360; 
elseif(err<-180)   
     err = 360 + err;
     
end

== matlab function coord2ASV1UAV/Co-Ordinated Motion 2 ASV 1 UAV/Simulated Vehicle/Dynamics/Dynamics ==
  data: u input; u_dot output; v input; r input; tau_u input; tau_r input; v_dot output; r_dot output
function [u_dot,v_dot,r_dot] = fcn(u,v,r,tau_u,tau_r)

% Coefficients
m = 17; %kg
Iz = 1; %4.14;
X_u_dot = -20;
Y_v_dot = -30;%-1.3175;
N_r_dot = -8.69;% -0.5;
X_u = -0.2;
Y_v = -50; %-55.117;
N_r = -4.14; %-0.1
X_uu = -25;
Y_vv = -0.01;%-101.2776;
N_rr = -6.23; %-21

% Added Mass
mu = m - X_u_dot;
mv = m - Y_v_dot;
mr = Iz - N_r_dot;
muv = mu - mv;

% Hydrodynamic Damping
du = - X_u - X_uu*abs(u);
dv = - Y_v - Y_vv*abs(v);
dr = - N_r - N_rr*abs(r);

% State Derivatives
u_dot = 1/mu*(tau_u + mv*v*r - du*u);
v_dot = 1/mv*(- mu*u*r - dv*v);
r_dot = 1/mr*(tau_r + muv*u*v - dr*r);

== matlab function coord2ASV1UAV/Co-Ordinated Motion 2 ASV 1 UAV/ASV Reference Provider/Path Controller/Path Yaw Controller ==
  data: yawRef1 output; uRef input; dError input; errorInt input; error input; yawRef2 output; yawD input
function [yawRef1, yawRef2]  = yawController(uRef, dError, errorInt, error, yawD)
%number of vehicles
n = 2;

% Gain Values
K1 =  6.0; %yaw proportional
K2 =  10.0; %cross-track proportional
K3 =  0.0; %cross-track differential
K4 =  0.6; %integral

%assign matrices
yawDel = zeros(1,n);

    %loop through vehicles
    for i = 1:n
        %extract data
        yError     =    error(1,i);
        yawError   =    error(2,i);
        yError_dot =   dError(1,i);
        yInt       = errorInt(1,i);

        %provide delta term
        yawDel(1,i) = K1*yawError + K2*yError/uRef ...
                      + K3*yError_dot + K4*yInt;
    end   
    
%provide yawRef values (2 VEHICLES)
yawRef1 = + yawDel(1,1) + yawD(1,1);
yawRef2 = + yawDel(1,2) + yawD(1,2);

end

== matlab function coord2ASV1UAV/Co-Ordinated Motion 2 ASV 1 UAV/ASV Reference Provider/Path Controller/Process Path ==
  data: start input; yawD_i output; c_i output; finish input; n input
function [yawD_i, c_i] = fcn(start, finish ,n)
% INPUTS
% n     = vehicle ID no.
% start = [xs1, xs2,...,xsi;
%          ys1, ys2,...,ysi]
% end   = [xe1, xe2,...,xei;
%          ye1, ye2,...,yei]
% for i = {1,..,n} vehicles


% % desired yaw
% m1 = (finish(2,1) - start(2,1)) / (finish(1,1) - start(1,1));
% m2 = (finish(2,2) - start(2,2)) / (finish(1,2) - start(1,2));
% yawD1 = atand(m1);
% yawD2 = atand(m2);
% yawD_i = [yawD1, yawD2];
% 
% % y intercept
% c1 = start(2,1) - m1*start(1,1);
% c2 = start(2,2) - m2*start(1,2);
% c_i = [c1, c2];

n = 2;

%assign matrices
yawD_i = zeros(1,n);
c_i    = zeros(1,n);

%loop through vehicles
for i = 1:n

    %desired yaw
    m = (finish(2,i) - start(2,i)) / (finish(1,i) - start(1,i));
    yawD_i(1,i) = -atan2d((finish(2,i) - start(2,i)),(finish(1,i) - start(1,i))) + 90;

    %y intersection
    c_i(1,i)    = start(2,i) - m*start(1,i);
end
end

== matlab function coord2ASV1UAV/Co-Ordinated Motion 2 ASV 1 UAV/ASV Reference Provider/Path Controller/Path Error ==
  data: pos_i input; yaw_i input; yawD input; c_i input; error output
% ========================================= %
% Calculating the cross track error between %
% defined path line and current position    %
% ========================================= %

function error  = pathError(pos_i, yaw_i, yawD, c_i)

% ARGUMENTS %
% x          current x position
% y          current y position
% m          gradient (for y = mx + c)
% c          y offset (for y = mx + c)

% VARIABLES %
% xD, yD     closest points on line
% error      error in [x, y, yaw]'
% u          vector between desired and real paths 

%number of vehicles
n = 2;

%assign matrices
error    = zeros(2,n);

%function to minimize
    function u = lineDiff(xL)
        u = (xL - x)^2 + (m*xL + c - y)^2;
    end

%loop through vehicles
for i = 1:n
    
    %extract data
    x = pos_i(1,i);
    y = pos_i(2,i);
    m = tand(-yawD(1,i) + 90);
    if (abs(m) == Inf)
        m = 1000000;
    end
    c = c_i(1,i);    
    
    %desired position
    xD = fminbnd(@lineDiff,x-10,x+10);
    yD = m*xD + c;
    closestPoint = [xD,yD];

    %cross track error
%     e = sqrt(lineDiff(xD));
    e = sqrt((xD-x)^2 + (yD - y)^2);
    if y < (m*x + c)
        e = -e;
    end

    %yaw error
    yawErr = + yawD(1,i) - yaw_i(1,i);

    %combine error terms
    error(1,i) = e;
    error(2,i) = yawErr;

end
end

== matlab function coord2ASV1UAV/Co-Ordinated Motion 2 ASV 1 UAV/ASV Reference Provider/Start Controller/Decision Maker ==
  data: state1 input; decision output; state2 input
function decision = fcn(state1, state2)
% If both vehicles reach start point, decision = 1
    if (state1 > 0 && state2 > 0)
        decision = 1;
    else
        decision = 0;
    end
end

== matlab function coord2ASV1UAV/Co-Ordinated Motion 2 ASV 1 UAV/ASV Reference Provider/Start Controller/Start 1 ==
  data: yawRef output; x input; y input; uRef output; start input; finish input; ku parameter; ks parameter; state output
% % % START POINT CONTROLLER % % %
% Make vehicle reach desired point
% Orient vehicle in direction of path

function [yawRef, uRef, state] = wayPoint(x,y, start, finish, ku, ks)
    % Go to waypoint
    state = 0;

    % Margin of error
    e = 0.1;

    % Extract information from inputs
    point1 =  start(:,1);
    point2 = finish(:,1);

    xd1 = point1(1,1);
    yd1 = point1(2,1);

    xd2 = point2(1,1);
    yd2 = point2(2,1);

    % Distance to waypoint
    d = sqrt((x - xd1)^2 + (y - yd1)^2) - e;

    % Decide on action
    if (d < 0) % vehicle in desired region
        state = 1;
        uRef = 0;
        % point in direction of path
        yawRef = -atan2d((yd2-yd1),(xd2-xd1)) + 90;
    else % vehicle outwith region
        uRef = ku*asin(d /(abs(d)+ks))*2/pi;
        yawRef = -atan2d((yd1-y), (xd1-x)) + 90;
    end
end

== matlab function coord2ASV1UAV/Co-Ordinated Motion 2 ASV 1 UAV/Coordination/Co-Ordination Controller ==
  data: n input; vcorr1 output; pos_i input size=[2,2]; start input; finish input; pathType input; vcorr2 output; ks parameter; ksync parameter; decision input
%% COORDINATION CONTROLLER
% ----INPUTS---- %
% VEHICLES
%  n = number of vehicles

% CURRENT STATE
% pos_i    = [x1, x2, ..., xn;
%             y1, y2, ..., yn];
% where i  = {1,n}
% decision = 1 ; if coordination required
% decision = 0 ; otherwise

% PATH DEFINITION
% point = [xs1, xs2, ..., xsn;
%          ys1, ys2, ..., ysn];
% where s is start, f is finish
% number denotes vehicle number
%
% pathType
% 0: line
% 1: arc

% ----OUTPUT---- %
% vcorr = [vcorr1, vcorr2, ..., vcorrn] (m/s)
%% IMPLEMENTATION
function [vcorr1,vcorr2]  = coOrd(n, pos_i, start, finish, pathType, ks, ksync, decision)
% Check whether in path following mode
if decision > 0
    % Check inputs valid
    [a,b] = size(start);
    [c,d] = size(finish);
    if (a ~= 2 || b ~= n || c ~= 2 || d ~= n )
        disp('path variable invalid')
    end

    % establish matrice sizes
    gamma  = zeros(1,n);
    gammaE = zeros(1,n);
    vcorr  = zeros(1,n);
    length = zeros(1,n);

    % CALCULATE PATH LENGTH VARIABLES
    switch pathType
        % STRAIGHT LINE
        case 0
            for i = 1:n
                length(1,i) = sqrt((finish(1,i)-start(1,i))^2 + (finish(2,i)-start(2,i)^2));
                % coordination state
                gamma(1,i) = sum(1/length(1,i) * (pos_i(:,i) - start(:,i)));
            end
        % ARC
        case 1
            for i = 1:n
                % midpoint
                M = [(start(1,i)+finish(1,i))/2, (start(2,i)+finish(2,i))/2];
                % gradient
                m = (finish(2,i)-start(2,i))/(finish(1,i)-start(1,i));
                grad = -atan(m);
                % Transformation
                T = [cos(grad), -sin(grad), -M(1);
                    sin(grad),  cos(grad), -M(2);
                    0,          0,          1  ];
                %position
                posHold = T*[pos_i(:,i);1];
                pos_i(:,i) = posHold(1:2,1);
                %start
                startHold = T*[start(:,i);1];
                start(:,i) = startHold(1:2,1);
                %finish
                finishHold = T*[finish(:,i);1];
                finish(:,i) = finishHold(1:2,1);
                %length
                length(1,i) = pi/2 * sqrt((finish(1,i)-start(1,i))^2 + (finish(2,i)-start(2,i)^2));
                % coordination state
                gamma(1,i) = sum(1/length(1,i) * (pos_i(:,i) - start(:,i)));
            end
        otherwise
            disp('invalid path type')
    end

    % COORDINATION
    for i = 1:n
        % coordination error
        gammaE(1,i) = gamma(1,i) - 1/n * sum(gamma);
        % correction velocity
        vcorr(1,i) = -ksync * asin(gammaE(1,i) / (abs(gammaE(1,i)) + ks)) * 2/pi;
    end

    vcorr1 = vcorr(1,1);
    vcorr2 = vcorr(1,2);
else
    vcorr1 = 0;
    vcorr2 = 0;
end

end

== matlab function coord2ASV1UAV/Co-Ordinated Motion 2 ASV 1 UAV/ASV Reference Provider/Start Controller/Start 2 ==
  data: yawRef output; x input; y input; uRef output; start input; finish input; ku parameter; ks parameter; state output
% % % START POINT CONTROLLER % % %
% Make vehicle reach desired point
% Orient vehicle in direction of path

function [yawRef, uRef,state] = wayPoint(x,y, start, finish, ku, ks)   
    % Go to waypoint
    state = 0;
    
    % Margin of error
    e = 0.1;
    
    % Extract information from inputs
    point1 =  start(:,2);
    point2 = finish(:,2);
    
    xd1 = point1(1,1); 
    yd1 = point1(2,1);
    
    xd2 = point2(1,1); 
    yd2 = point2(2,1);
    
    % Distance to waypoint
    d = sqrt((x - xd1)^2 + (y - yd1)^2) - e;
    
    % Decide on action
    if (d < 0) % vehicle in desired region
        state = 1;
        uRef = 0;
        % point in direction of path
        yawRef = -atan2d((yd2-yd1),(xd2-xd1)) + 90;
    else % vehicle outwith region
        uRef = ku*asin(d /(abs(d)+ks))*2/pi;
        yawRef = -atan2d((yd1-y), (xd1-x)) + 90;
    end
end

== matlab function coord2ASV1UAV/Co-Ordinated Motion 2 ASV 1 UAV/ASV Reference Provider/Waypoint Controller/Waypoint Controller ==
  data: yawRef1 output; uRef1 output; pos_i input; yawRef2 output; uRef2 output; start input; finish input; state output; ku parameter; ks parameter
function [yawRef1, uRef1, yawRef2, uRef2, state] = wayPoint(pos_i, start, finish, ku, ks)
    state = 0;
    % margin
    e = 0.1;
    % number of vehicles
    n = 2;
    
    % assign matrices
    yawRef =    zeros(1,n);
    uRef =      zeros(1,n);
    d =         zeros(1,n);
    stateHold = zeros(1,n);
    
    % loop through vehicles
    for i = 1:n

        % extract information
        x0 =  start(1,i);
        y0 =  start(2,i);
        x1 = finish(1,i);
        y1 = finish(2,i);
        
        x =   pos_i(1,i);
        y =   pos_i(2,i);

        % distance to waypoint
        d(1,i) = sqrt((x - x0)^2 + (y - y0)^2) - e;

        % decide on action
        if (d(1,i) < 0)
            stateHold(1,i) = 1;
            uRef(1,i) = 0;
            yawRef(1,i) = atan2d((y1-y0),(x1-x0));
        else
            uRef(1,i) = ku*asin(d /(abs(d)+ks))*2/pi;
            yawRef(1,i) = - atan2d((y0-y),(x0-x)) + 90;
        end
        
        % change state
        if (all(stateHold))
            state = 1;
        end
            
    end
    
    % Provide references
    yawRef1 = yawRef(1,1);
    yawRef2 = yawRef(1,2);
    
    uRef1 = uRef(1,1);
    uRef2 = uRef(1,2);
end

== matlab function coord2ASV1UAV/Co-Ordinated Motion 2 ASV 1 UAV/Simulated Vehicle/Dynamics/Kinematics ==
  data: u input; x_dot output; v input; r input; yaw input; y_dot output; yaw_dot output
function [x_dot,y_dot,yaw_dot] = fcn(u,v,r,yaw)

y_dot = u*cos(yaw) - v*sin(yaw);
x_dot = u*sin(yaw) + v*cos(yaw);
yaw_dot = r;

== matlab function coord2ASV1UAV/Co-Ordinated Motion 2 ASV 1 UAV/Simulated Vehicle/Heading Controller/MATLAB Function ==
  data: err output; yawRef input; yawIn input
function err = fcn(yawRef,yawIn)
%error term
err = yawRef - yawIn;

%normalize
if(err>180) 
     err = err - 360; 
elseif(err<-180)   
     err = 360 + err;
     
end

== matlab function coord2ASV1UAV/Co-Ordinated Motion 2 ASV 1 UAV/Simulated Vehicle/Moter Power/MATLAB Function ==
  data: dmHead input; cmSpeed input; Pm output; Sm output
function [Pm,Sm] = fcn(dmHead,cmSpeed)

Cm_sqr = cmSpeed;
Dm_sqr = dmHead;

Pm = round(sqrt(abs(Cm_sqr+Dm_sqr))*sign(Cm_sqr+Dm_sqr));
Sm = round(sqrt(abs(Cm_sqr-Dm_sqr))*sign(Cm_sqr-Dm_sqr));

== matlab function coord2ASV1UAV/Co-Ordinated Motion 2 ASV 1 UAV/Simulated Vehicle/Speed Controller1/u Speed from Estimates ==
  data: vx input; cm output; vy input; yaw input; Uref input; int output; intOld input; Kp parameter; Ki parameter; KSat parameter
function [cm,int] = ExtractSpeed(vx,vy,yaw,Uref,intOld,Kp, Ki, KSat)

% Kp = 60;
% Ki = 2;
% KSat = 60;
 
u = vx*sind(yaw) + vy*cosd(yaw);
err = u - Uref;
int = intOld + err;

cm = - Kp*err - Ki*int;

if(abs(cm) >= KSat)
   cm = KSat*sign(cm); 
   int = intOld;
end

== matlab function coord2ASV1UAV/Co-Ordinated Motion 2 ASV 1 UAV/ASV Reference Provider/Start Controller/MATLAB Function1 ==
  data: pos_i input; x1 output; y1 output; x2 output; y2 output
function [x1,y1,x2,y2] = fcn(pos_i)
% Vehicle 1
x1 = pos_i(1,1);
y1 = pos_i(2,1);
% Vehicle 2
x2 = pos_i(1,2);
y2 = pos_i(2,2);
end

== matlab function coord2ASV1UAV/Co-Ordinated Motion 2 ASV 1 UAV/Signal Compiler/MATLAB Function ==
  data: x1 input; pos_i output; y1 input; yaw1 input; x2 input; y2 input; yaw2 input; yaw_i output size=[1 2]
% % % 2 VEHICLES SIGNAL COMPILER % % %

function [pos_i, yaw_i] = compilePositions(x1, y1, yaw1, x2, y2, yaw2)
    pos_i = [x1,x2;y1,y2];
    yaw_i = [yaw1,yaw2];
end
